simulink model "verify_Fan_Const_mdl"  (R2018b)
settings: Solver=ode45  StartTime=0.0  StopTime=240  MaxStep=1  RelTol=1e-3  EnableMultiTasking=on
libraries: carnot x2, simulink x1
settings Model: Creator=drhf  LastModifiedBy=drhf
settings DataIOCC: SaveFormat=Array  SignalLoggingSaveFormat=ModelDataLogs
settings OptimizationCC: ExpressionDepthLimit=2147483647  LifeSpan=inf
settings DebuggingCC: UnderspecifiedInitializationDetection=Classic  MergeDetectMultiDrivingBlocksExec=none  SolverPrmCheckMsg=warning  FcnCallInpInsideContextMsg=warning  StateNameClashWarn=warning  SFUnexpectedBacktrackingDiag=warning  SFNoUnconditionalDefaultTransitionDiag=warning  SFExecutionAtInitializationDiag=none
settings HardwareCC: ProdBitPerPointer=32  ProdBitPerSizeT=32  ProdBitPerPtrDiffT=32  ProdLargestAtomicFloat=None  ProdIntDivRoundTo=Undefined  ProdEndianess=Unspecified  ProdWordSize=32  ProdHWDeviceType=32-bit Generic
settings ModelReferenceCC: PropagateSignalLabelsOutOfModel=off
settings SFSimCC: SimUseLocalCustomCode=off
settings RTWCC: RTWUseLocalCustomCode=off
settings CodeAppCC: StateflowObjectComments=on
settings GRTTargetCC: TargetLangStandard=C89/C90 (ANSI)  GeneratePreprocessorConditionals=Disable all  CombineOutputUpdateFcns=off  GRTInterface=on
settings ConfigComp: CovMetricSettings=dw  CovHtmlReporting=on  CovSaveCumulativeToWorkspaceVar=on  CovSaveSingleToWorkspaceVar=on  CovExternalEMLEnable=off

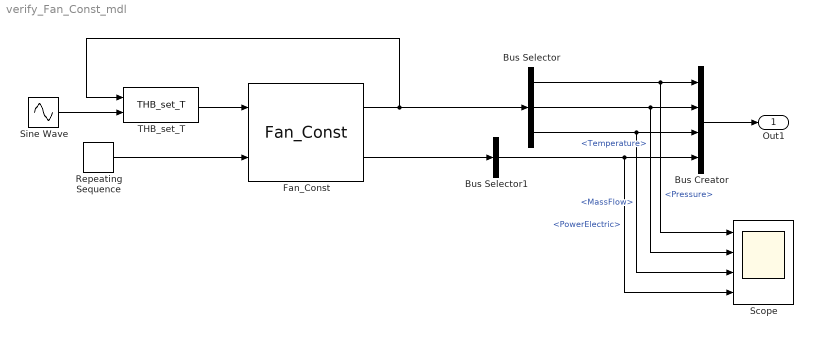
== system verify_Fan_Const_mdl ==
  Bus Creator : BusCreator  Inputs=4
  Bus Selector : BusSelector  OutputSignals=Pressure,Temperature,MassFlow
  Bus Selector1 : BusSelector  OutputSignals=PowerElectric
  Fan_Const : carnot/Hydraulics/Fan_Const  Vdotmax=1000  dia=0.5  p0=101300  mix=0.01  Tini=20  UA=3  mcp=1000  e0=10  e1=10  e2=-1
      settings: SourceProductName=Carnot
  Repeating Sequence : simulink/Sources/Repeating Sequence  rep_seq_t=[0 120 240]  rep_seq_y=[0 1 0]
  Scope : Scope  NumInputPorts=4
  Sine Wave : Sin  Amplitude=5  Bias=20  Frequency=2*pi/240  SampleTime=0
  THB_set_T : carnot/Source/Simple/THB_set_T
      settings: SourceProductName=Carnot
  Out1 : Outport
  wires:
  Bus Creator/1 -> Out1/1
  Bus Selector/3 -> Scope/3, Bus Creator/3  "<MassFlow>"
  Repeating Sequence/1 -> Fan_Const/2
  Fan_Const/1 -> THB_set_T/1, Bus Selector/1
  Fan_Const/2 -> Bus Selector1/1
  Bus Selector/1 -> Scope/1, Bus Creator/1  "<Pressure>"
  Bus Selector/2 -> Scope/2, Bus Creator/2  "<Temperature>"
  Sine Wave/1 -> THB_set_T/2
  THB_set_T/1 -> Fan_Const/1
  Bus Selector1/1 -> Scope/4, Bus Creator/4  "<PowerElectric>"
